simulink model "dx_hand_model_rai3"  (R2017b)
settings: Solver=ode3  StartTime=0.0  StopTime=inf  FixedStep=0.01  RelTol=1e-3  EnableMultiTasking=on
InitFcn:
  | cutFreq = 0.1; % T
  | sampleTime = 0.01;
  | filt = tf(1,[cutFreq 1]);
  | filt = c2d(filt,sampleTime);
  | 
  | cutFreq2 = 1;
  | filt2 = tf(1,[cutFreq2 1]);
  | filt2 = c2d(filt2,sampleTime);
  | 
  | update_param = 2;
  | 
  | ampliFactor = 1.60;
  | ampliFactorMiddle = 2.00;
  | ampliFactorDistal = 1;
  | 
  | % Set Hand Address
  | RightHandAddress = '10.24.4.91';
  | Verosim = '10.100.39.22'
  | LeftHandAddress = '10.24.4.90'
  | 
  | max_force = 12; % Newton
model workspace (MAT data in the model file):
  SL_ROS_VariableLengthArrays_MaxSizes.CommonInfo.ArrayTruncateAction = 'EmitWarning'
  SL_ROS_VariableLengthArrays_MaxSizes.MsgTypeMap = containers.Map
  SL_ROS_VariableLengthArrays_MaxSizes.MsgTypeMap.serialization.keys = {'std_msgs/Float32MultiArray'}
  SL_ROS_VariableLengthArrays_MaxSizes.MsgTypeMap.serialization.values{1}.PropertyName = 'Data'
  SL_ROS_VariableLengthArrays_MaxSizes.MsgTypeMap.serialization.values{1}.DataType = 'single'
  SL_ROS_VariableLengthArrays_MaxSizes.MsgTypeMap.serialization.values{1}.MaxLength = 2
  SL_ROS_VariableLengthArrays_MaxSizes.MsgTypeMap.serialization.uniformity = 0
  SL_ROS_VariableLengthArrays_MaxSizes.MsgTypeMap.serialization.keyType = 'char'
  SL_ROS_VariableLengthArrays_MaxSizes.MsgTypeMap.serialization.valueType = 'any'
libraries: robotlib x134, simulink_extras x28, simulink x16, dspnetwork x5, etargetslib x4
(part 1 of 19)
settings Model: Creator=Centauro  LastModifiedBy=exo-hand
settings DataIOCC: LimitDataPoints=on  SaveFormat=Array
settings OptimizationCC: PassReuseOutputArgsThreshold=0  MaxStackSize=64
settings DebuggingCC: ParameterTunabilityLossMsg=error  SFUnexpectedBacktrackingDiag=warning  SFNoUnconditionalDefaultTransitionDiag=warning  SFExecutionAtInitializationDiag=none
settings HardwareCC: ProdBitPerPointer=32  ProdBitPerSizeT=32  ProdBitPerPtrDiffT=32  ProdLargestAtomicFloat=None  ProdIntDivRoundTo=Undefined  ProdEndianess=Unspecified  ProdWordSize=32  ProdHWDeviceType=Generic->Unspecified (assume 32-bit Generic)  UseEmbeddedCoderFeatures=off
settings ModelReferenceCC: PropagateSignalLabelsOutOfModel=off
settings SFSimCC: MATLABDynamicMemAlloc=off
settings RTWCC: SystemTargetFile=ert.tlc  HardwareBoard=Robot Operating System (ROS)  TemplateMakefile=ert_default_tmf  GenerateReport=on  Toolchain=Catkin  LaunchReport=on  TargetLang=C++
settings CodeAppCC: ForceParamTrailComments=on  OperatorAnnotations=on
settings ERTTargetCC: ERTCustomFileBanners=off  SupportContinuousTime=on  SupportNonInlinedSFcns=on  RemoveResetFunc=off  ModelStepFunctionPrototypeControlCompliant=off
settings ConfigComp: CovMetricSettings=dw  CovHtmlReporting=on  CovSaveCumulativeToWorkspaceVar=on  CovSaveSingleToWorkspaceVar=on  CovExternalEMLEnable=off

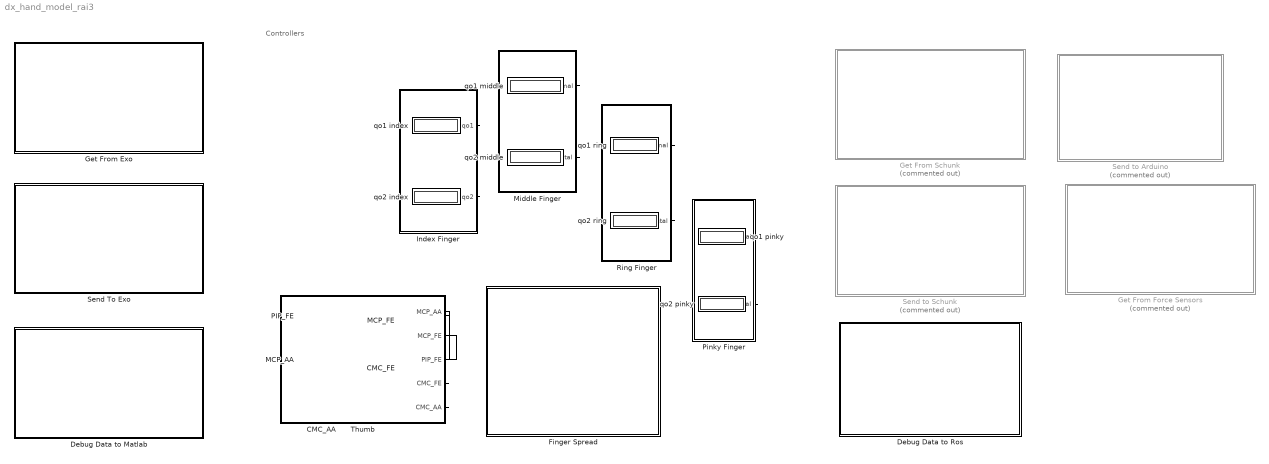
== system dx_hand_model_rai3 ==
  note: Controllers
  CMC_AA : Display
  CMC_FE : Display
  Debug Data to Matlab : Subsystem
  Debug Data to Ros : Subsystem
  Finger Spread : Subsystem
  Get From Exo : Subsystem
  Get From Force Sensors : Subsystem  Commented=on
  Get From Schunk : Subsystem  Commented=on
  Index Finger : Subsystem
  MCP_AA : Display
  MCP_FE : Display
  Middle Finger : Subsystem
  PIP_FE : Display
  Pinky Finger : Subsystem
  "Ring Finger " : Subsystem
  Send To Exo : Subsystem
  Send to Arduino : Subsystem  Commented=on
  Send to Schunk : Subsystem  Commented=on
  Thumb : Subsystem
  qo1 index : Display
  qo1 middle : Display
  qo1 pinky : Display
  qo1 ring : Display
  qo2 index : Display
  qo2 middle : Display
  qo2 pinky : Display
  qo2 ring : Display
  wires:
  Pinky Finger/1(proximal) -> qo1 pinky/1
  "Ring Finger "/1(proximal) -> qo1 ring/1
  Index Finger/2("qo2 ") -> qo2 index/1
  Index Finger/1("qo1 ") -> qo1 index/1
  Middle Finger/2(distal) -> qo2 middle/1
  Middle Finger/1(proximal) -> qo1 middle/1
  Thumb/1(MCP_AA) -> MCP_AA/1
  Thumb/2(MCP_FE) -> MCP_FE/1
  Thumb/4(CMC_FE) -> CMC_FE/1
  Thumb/3(PIP_FE) -> PIP_FE/1
  Thumb/5(CMC_AA) -> CMC_AA/1
  "Ring Finger "/2(distal) -> qo2 ring/1
  Pinky Finger/2(distal) -> qo2 pinky/1

== system dx_hand_model_rai3/Debug Data to Matlab ==
  Constant : Constant
  Constant1 : Constant  Value=0
  Manual Switch : ManualSwitch
  Mux : Mux  Inputs=20
  Thumb Exo Structure : Subsystem
  wires:
  Manual Switch/1 -> Thumb Exo Structure/Enable
  Constant/1 -> Manual Switch/2
  Constant1/1 -> Manual Switch/1
  [thumb_i] -> Mux/11
  [thumb_g2] -> Mux/9
  [thumb_c] -> Mux/3
  [thumb_d] -> Mux/4
  [thumb_f] -> Mux/7
  [thumb_f1] -> Mux/6
  [thumb_h] -> Mux/10
  [thumb_b] -> Mux/2
  Mux/1 -> Thumb Exo Structure/1(In1)
  [thumb_j] -> Mux/12
  [thumb_CMC] -> Mux/1
  [thumb_e] -> Mux/5
  [thumb_g1] -> Mux/8
  [thumb_MCP] -> Mux/13
  [thumb_K] -> Mux/14
  [thumb_PIP] -> Mux/15
  [thumb_K2] -> Mux/16
  [thumb_s1] -> Mux/17
  [thumb_l_meta] -> Mux/18
  [thumb_s2] -> Mux/19
  [thumb_l_dist] -> Mux/20

== system dx_hand_model_rai3/Debug Data to Ros ==
  Send : Subsystem
  Vector Concatenate : Concatenate  NumInputs=5
  Vector Concatenate1 : Concatenate  NumInputs=5
  wires:
  Vector Concatenate/1 -> Send/1(to_exo)
  Vector Concatenate1/1 -> Send/2(from_exo)
  [SetHandIndexForce] -> Vector Concatenate/2
  [SetHandRingForce] -> Vector Concatenate/4
  [SetHandThumbForce] -> Vector Concatenate/1
  [SetHandMiddleForce] -> Vector Concatenate/3
  [SetHandPinkyForce] -> Vector Concatenate/5
  [PinkyForce] -> Vector Concatenate1/5
  [RingForce] -> Vector Concatenate1/4
  [MiddleForce] -> Vector Concatenate1/3
  [IndexForce] -> Vector Concatenate1/2
  [ThumbForce] -> Vector Concatenate1/1

== system dx_hand_model_rai3/Finger Spread ==
  Constant : Constant  Value=0.0  OutDataTypeStr=single
  Constant1 : Constant  Value=0.15  OutDataTypeStr=single
  Display : Display
  MATLAB Function : MATLAB Function  TreatAsAtomicUnit=on
  Manual Switch : ManualSwitch  CurrentSetting=0
  Mux : Mux  Inputs=2
  Sum : Sum  Inputs=|++
  calibration1 : Subsystem
  tag scope: SchunkFingerSpread=global
  wires:
  [IndexSpreadRotPot] -> calibration1/1(In1), MATLAB Function/1(u)
  Constant/1 -> Manual Switch/2
  MATLAB Function/1(y) -> Manual Switch/1
  calibration1/1(Out1) -> Mux/2, MATLAB Function/2(calib)
  Mux/1 -> Display/1
  Manual Switch/1 -> Sum/1
  Sum/1 -> Mux/1, [SchunkFingerSpread]
  Constant1/1 -> Sum/2

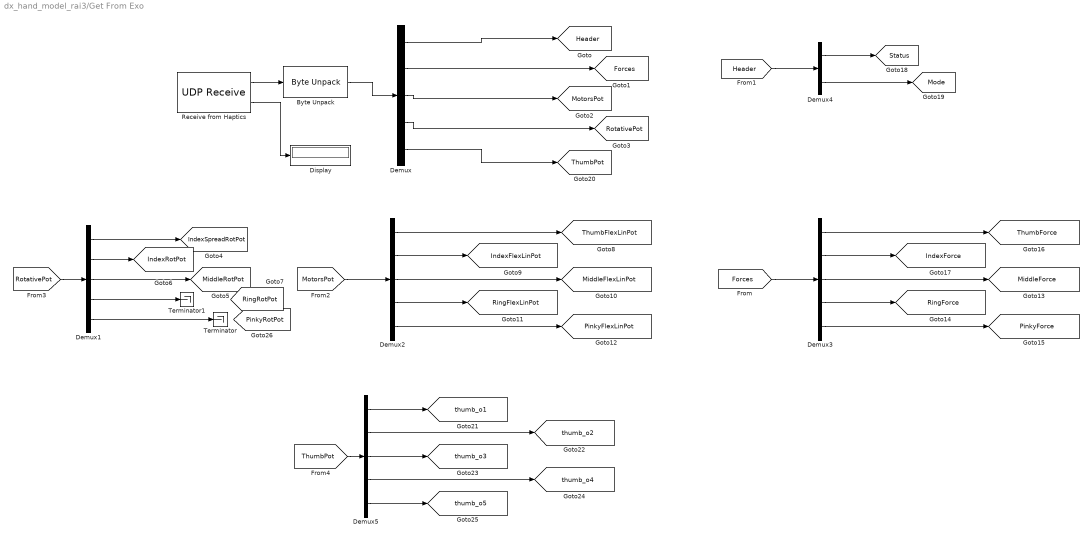
== system dx_hand_model_rai3/Get From Exo ==
  Byte Unpack : etargetslib/Byte Unpack  dimensions={[22]}  datatypes={'single'}  byteAlign=1
  Demux : Demux  Outputs=[2, 5, 5, 5,5]
  Demux{1..3,5} (4 alike) : Demux  Outputs=5
  Demux4 : Demux  Outputs=2
  Display : Display
  Receive from Haptics : dspnetwork/UDP Receive  localURL='0.0.0.0'  localPort=15001  remoteURL='0.0.0.0'  remotePort=-1  recvBufferSize=22*4  dims=22*4  signalDatatype=uint8  isVarSize=off  showBlockingTime=on  blockingTime=inf  sampletime=0.01  blockPlatform=HOST
      settings: SourceProductName=DSP System Toolbox  SourceProductBaseCode=DS
  Terminator : Terminator
  Terminator1 : Terminator
  tag scope: Forces=global, Header=global, IndexFlexLinPot=global, IndexForce=global, IndexRotPot=global, IndexSpreadRotPot=global, MiddleFlexLinPot=global, MiddleForce=global, MiddleRotPot=global, Mode=global, MotorsPot=global, PinkyFlexLinPot=global, PinkyForce=global, PinkyRotPot=global, RingFlexLinPot=global, RingForce=global, RingRotPot=global, RotativePot=global, Status=global, ThumbFlexLinPot=global, ThumbForce=global, ThumbPot=global, thumb_o1=global, thumb_o2=global, thumb_o3=global, thumb_o4=global, thumb_o5=global
  wires:
  Demux/3 -> [MotorsPot]
  Demux/1 -> [Header]
  Demux/4 -> [RotativePot]
  Demux/2 -> [Forces]
  Receive from Haptics/2 -> Display/1
  [RotativePot] -> Demux1/1
  Demux1/2 -> [IndexRotPot]
  Demux1/3 -> [MiddleRotPot]
  Demux1/4 -> Terminator1/1
  Demux1/5 -> Terminator/1
  Demux1/1 -> [IndexSpreadRotPot]
  Demux2/1 -> [ThumbFlexLinPot]
  Demux2/2 -> [IndexFlexLinPot]
  [MotorsPot] -> Demux2/1
  Demux2/3 -> [MiddleFlexLinPot]
  Demux2/4 -> [RingFlexLinPot]
  Demux2/5 -> [PinkyFlexLinPot]
  Demux3/1 -> [ThumbForce]
  Demux3/2 -> [IndexForce]
  [Forces] -> Demux3/1
  Demux3/3 -> [MiddleForce]
  Demux3/4 -> [RingForce]
  Demux3/5 -> [PinkyForce]
  [Header] -> Demux4/1
  Demux4/1 -> [Status]
  Demux4/2 -> [Mode]
  Byte Unpack/1 -> Demux/1
  Receive from Haptics/1 -> Byte Unpack/1
  Demux/5 -> [ThumbPot]
  [ThumbPot] -> Demux5/1
  Demux5/1 -> [thumb_o1]
  Demux5/2 -> [thumb_o2]
  Demux5/3 -> [thumb_o3]
  Demux5/4 -> [thumb_o4]
  Demux5/5 -> [thumb_o5]

== system dx_hand_model_rai3/Get From Force Sensors ==
  Currents : Subsystem

== system dx_hand_model_rai3/Get From Schunk ==
  Currents : Subsystem
  Get positions : Subsystem

== system dx_hand_model_rai3/Index Finger ==
  note: To Schunk
  note: To Exo
  Active : Subsystem
  Choose : Subsystem
  Display : Display
  Force : Subsystem
  Jacobian Calculation : Subsystem
  Pose Generator : Subsystem
  Position : Subsystem
  Pre-Proc : Subsystem
  Send Position : Subsystem
  setGain2 : Subsystem
  "qo1 " : Outport
  "qo2 " : Outport  Port=2
  tag scope: IndexForceReference=global
  wires:
  Pose Generator/1(Pose) -> Send Position/1(Pose), Jacobian Calculation/1(Pose)
  Pose Generator/2(Sensors) -> Jacobian Calculation/2(Sensor)
  Pose Generator/3("Measurements ") -> Jacobian Calculation/3(Measurements)
  Send Position/1(qo1) -> "qo1 "/1
  Send Position/2("qo2 ") -> "qo2 "/1
  Position/1(rate) -> Choose/1(pos)
  Force/1(Feedforward Force) -> Choose/2(force)
  Choose/1(out) -> setGain2/1(in)
  setGain2/1(out) -> Display/1, Active/1(in)
  Jacobian Calculation/1(Jac) -> Pre-Proc/1(in)
  Pre-Proc/1(out) -> Force/1(Jacobian), Position/1(Jacobian)
  Active/1(out) -> [IndexForceReference]

== system dx_hand_model_rai3/Middle Finger ==
  note: To Schunk
  note: To Exo
  Active : Subsystem
  Choose : Subsystem
  Demux : Demux  Outputs=8
  Display2 : Display
  Jacobian Calculation : Subsystem
  Pose Generator : Subsystem
  Position-Force Architecture : Subsystem
  Position-Position : Subsystem
  Pre-Proc : Subsystem
  Radians to Degrees : simulink_extras/Transformations/Radians to Degrees
  Radians to Degrees1 : simulink_extras/Transformations/Radians to Degrees
  setGain : Subsystem
  setGain1 : Subsystem
  setGain2 : Subsystem
  proximal : Outport
  distal : Outport  Port=2
  tag scope: MiddleForceReference=global, SchunkMiddleFingerDistal=global, SchunkMiddleFingerProximal=global
  wires:
  Demux/2 -> Radians to Degrees/1, setGain1/1(in)
  Pose Generator/1(Pose) -> Demux/1, Jacobian Calculation/1(Pose)
  Pose Generator/2(Sensors) -> Jacobian Calculation/2(Sensor)
  Pose Generator/3(Measurements) -> Jacobian Calculation/3(Measurements)
  Demux/1 -> Radians to Degrees1/1, setGain/1(in)
  Radians to Degrees1/1 -> proximal/1
  Radians to Degrees/1 -> distal/1
  Position-Force Architecture/1(Feedforward Force) -> Choose/2(force)
  Jacobian Calculation/1(Jacobian) -> Pre-Proc/1(in)
  Pre-Proc/1(out) -> Position-Position/1(Jacobian), Position-Force Architecture/1(Jacobian)
  setGain2/1(out) -> Display2/1, Active/1(in)
  Position-Position/1(rate) -> Choose/1(pos)
  setGain/1(out) -> [SchunkMiddleFingerProximal]
  setGain1/1(out) -> [SchunkMiddleFingerDistal]
  Choose/1(out) -> setGain2/1(in)
  Active/1(out) -> [MiddleForceReference]

== system dx_hand_model_rai3/Pinky Finger ==
  note: To Exo
  note: To Schunk
  Active : Subsystem
  Choose : Subsystem
  Choose_ : Subsystem
  Demux : Demux  Outputs=8
  Display2 : Display
  Gain Aggiustato : Gain  Gain=50/1024
  Gain1 : Gain  Gain=0.98/40
  Jacobian Calculation : Subsystem
  Pose Generator : Subsystem
  Position-Force Architecture : Subsystem
  Position-Position : Subsystem
  Pre-Proc : Subsystem
  Radians to Degrees : simulink_extras/Transformations/Radians to Degrees
  Radians to Degrees1 : simulink_extras/Transformations/Radians to Degrees
  setGain : Subsystem
  setGain1 : Subsystem
  setGain2 : Subsystem
  proximal : Outport
  distal : Outport  Port=2
  tag scope: PinkyForceReference=global, SchunkPinkyFinger=global, SchunkPinkyFingerDistal=global, SchunkPinkyFingerProximal=global
  wires:
  [PinkyFlexLinPot] -> Gain Aggiustato/1
  Gain1/1 -> Choose/2(empiric)
  Gain Aggiustato/1 -> Gain1/1
  Jacobian Calculation/1(Jacobian) -> Pre-Proc/1(in)
  Position-Force Architecture/1(Feedforward Force) -> Choose_/2(force)
  Pose Generator/2(Sensors) -> Jacobian Calculation/2(Sensor)
  Choose_/1(out) -> setGain2/1(in)
  Pose Generator/3(Measurements) -> Jacobian Calculation/3(Measurements)
  Demux/2 -> Radians to Degrees/1, setGain1/1(in)
  Position-Position/1(rate) -> Choose_/1(pos)
  Radians to Degrees/1 -> distal/1
  Radians to Degrees1/1 -> proximal/1
  setGain2/1(out) -> Display2/1, Active/1(in)
  setGain1/1(out) -> [SchunkPinkyFingerDistal]
  setGain/1(out) -> Choose/1(theoretical), [SchunkPinkyFingerProximal]
  Pre-Proc/1(out) -> Position-Position/1(Jacobian), Position-Force Architecture/1(Jacobian)
  Demux/1 -> Radians to Degrees1/1, setGain/1(in)
  Pose Generator/1(Pose) -> Demux/1, Jacobian Calculation/1(Pose)
  Active/1(out) -> [PinkyForceReference]
  Choose/1(out) -> [SchunkPinkyFinger]

== system dx_hand_model_rai3/Ring Finger  ==
  note: To Schunk
  note: To Exo
  Active : Subsystem
  Choose : Subsystem
  Choose_ : Subsystem
  Demux : Demux  Outputs=8
  Display2 : Display
  Gain Aggiustato : Gain  Gain=50/1024
  Gain1 : Gain  Gain=0.98/25
  Jacobian Calculation : Subsystem
  Pose Generator : Subsystem
  Position-Force Architecture : Subsystem
  Position-Position : Subsystem
  Pre-Proc : Subsystem
  Radians to Degrees : simulink_extras/Transformations/Radians to Degrees
  Radians to Degrees1 : simulink_extras/Transformations/Radians to Degrees
  setGain : Subsystem
  setGain1 : Subsystem
  setGain2 : Subsystem
  proximal : Outport
  distal : Outport  Port=2
  tag scope: RingForceReference=global, SchunkRingFinger=global, SchunkRingFingerDistal=global, SchunkRingFingerProximal=global
  wires:
  [RingFlexLinPot] -> Gain Aggiustato/1
  Gain Aggiustato/1 -> Gain1/1
  Gain1/1 -> Choose/2(empiric)
  Radians to Degrees1/1 -> proximal/1
  Position-Position/1(rate) -> Choose_/1(pos)
  Pose Generator/2(Sensors) -> Jacobian Calculation/2(Sensor)
  Choose_/1(out) -> setGain2/1(in)
  Radians to Degrees/1 -> distal/1
  setGain1/1(out) -> [SchunkRingFingerDistal]
  Pose Generator/1(Pose) -> Demux/1, Jacobian Calculation/1(Pose)
  setGain/1(out) -> Choose/1(theoretical), [SchunkRingFingerProximal]
  Position-Force Architecture/1(Feedforward Force) -> Choose_/2(force)
  Pose Generator/3(Measurements) -> Jacobian Calculation/3(Measurements)
  Pre-Proc/1(out) -> Position-Position/1(Jacobian), Position-Force Architecture/1(Jacobian)
  Demux/2 -> Radians to Degrees/1, setGain1/1(in)
  setGain2/1(out) -> Display2/1, Active/1(in)
  Jacobian Calculation/1(Jacobian) -> Pre-Proc/1(in)
  Demux/1 -> Radians to Degrees1/1, setGain/1(in)
  Active/1(out) -> [RingForceReference]
  Choose/1(out) -> [SchunkRingFinger]

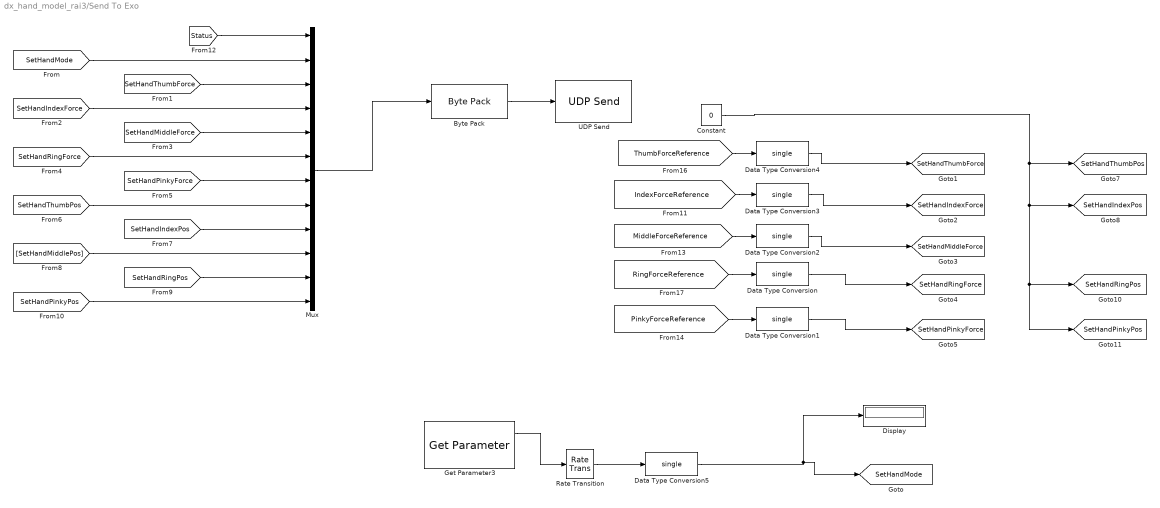
== system dx_hand_model_rai3/Send To Exo ==
  Byte Pack : etargetslib/Byte Pack  datatypes={'single'}  byteAlign=1
  Constant : Constant  Value=0  OutDataTypeStr=single
  Data Type Conversion{,1..5} (6 alike) : DataTypeConversion  OutDataTypeStr=single
  Display : Display
  Get Parameter3 : robotlib/Get Parameter  SourceLibraryInfo=This block requires Robotics System Toolbox  ParameterSource=Specify your own  ParameterName=/hand_exo/mode  ParameterType=double  ParameterMaxArrayLength=16  ParameterInitialValue=3.0  SampleTime=update_param  ShowErrorCodeOutput=on  ModelName=dx_hand_model_rai3  BlockId=ParamGet_dx_hand_model_rai3_2544
      settings: SourceProductName=Robotics System Toolbox  SourceProductBaseCode=RO
  Mux : Mux  Inputs=12
  Rate Transition : RateTransition
  UDP Send : dspnetwork/UDP Send  remoteURL=RightHandAddress  remotePort=12000  localURL='0.0.0.0'  localPortSource=Automatically determine  localPort=-1  sampletime=-1  blockPlatform=HOST  separateLengthPort=0
      settings: SourceProductName=DSP System Toolbox  SourceProductBaseCode=DS
  tag scope: SetHandIndexForce=global, SetHandIndexPos=global, SetHandMiddleForce=global, SetHandMode=global, SetHandPinkyForce=global, SetHandPinkyPos=global, SetHandRingForce=global, SetHandRingPos=global, SetHandThumbForce=global, SetHandThumbPos=global
  wires:
  Byte Pack/1 -> UDP Send/1
  [SetHandMode] -> Mux/2
  [SetHandThumbForce] -> Mux/3
  [SetHandIndexForce] -> Mux/4
  [SetHandRingForce] -> Mux/6
  [SetHandMiddleForce] -> Mux/5
  [SetHandPinkyForce] -> Mux/7
  [SetHandThumbPos] -> Mux/8
  [SetHandIndexPos] -> Mux/9
  [SetHandMiddlePos] -> Mux/10
  [SetHandRingPos] -> Mux/11
  [SetHandPinkyPos] -> Mux/12
  [Status] -> Mux/1
  [ThumbForceReference] -> Data Type Conversion4/1
  [RingForceReference] -> Data Type Conversion/1
  [PinkyForceReference] -> Data Type Conversion1/1
  [MiddleForceReference] -> Data Type Conversion2/1
  [IndexForceReference] -> Data Type Conversion3/1
  Constant/1 -> [SetHandThumbPos], [SetHandIndexPos], [SetHandRingPos], [SetHandPinkyPos]
  Mux/1 -> Byte Pack/1
  Data Type Conversion/1 -> [SetHandRingForce]
  Data Type Conversion1/1 -> [SetHandPinkyForce]
  Data Type Conversion2/1 -> [SetHandMiddleForce]
  Data Type Conversion3/1 -> [SetHandIndexForce]
  Data Type Conversion4/1 -> [SetHandThumbForce]
  Get Parameter3/1 -> Rate Transition/1
  Data Type Conversion5/1 -> [SetHandMode], Display/1
  Rate Transition/1 -> Data Type Conversion5/1

== system dx_hand_model_rai3/Send to Arduino ==
  Constant : Constant  Value=180
  Data Type Conversion2 : DataTypeConversion  OutDataTypeStr=uint8
  Display : Display
  Filt 4 : DiscreteTransferFcn  Numerator=filt.Numerator{1,1}  Denominator=filt.Denominator{1,1}  SampleTime=0.01
  Gain : Gain  Gain=180/60
  Radians to Degrees : simulink_extras/Transformations/Radians to Degrees
  Saturation : Saturate  UpperLimit=60  LowerLimit=0
  Sum : Sum  Inputs=|-+
  UDP Send : dspnetwork/UDP Send  remoteURL='10.24.4.20'  remotePort=9002  localURL='0.0.0.0'  localPortSource=Automatically determine  localPort=-1  sampletime=-1  blockPlatform=[]  separateLengthPort=0
      settings: SourceProductName=DSP System Toolbox  SourceProductBaseCode=DS
  wires:
  [SchunkIndexFingerProximal] -> Filt 4/1
  Filt 4/1 -> Radians to Degrees/1
  Radians to Degrees/1 -> Saturation/1
  Saturation/1 -> Gain/1
  Data Type Conversion2/1 -> Display/1, UDP Send/1
  Gain/1 -> Sum/1
  Sum/1 -> Data Type Conversion2/1
  Constant/1 -> Sum/2

== system dx_hand_model_rai3/Send to Schunk ==
  Enable : Subsystem  Commented=on
  Send data to Ros : Subsystem
  Signal Conditioning : Subsystem
  wires:
  Signal Conditioning/1(status) -> Send data to Ros/1(status)
  Signal Conditioning/3(data) -> Send data to Ros/2(data)

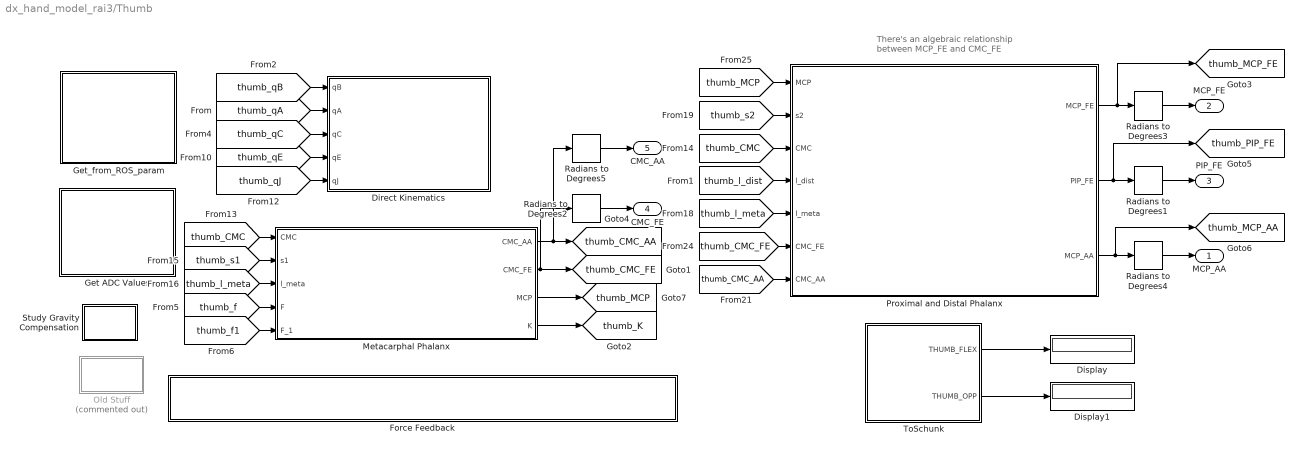
== system dx_hand_model_rai3/Thumb ==
  note: There's an algebraic relationship
      | between MCP_FE and CMC_FE
  Direct Kinematics : Subsystem
  Display : Display
  Display1 : Display
  Force Feedback : Subsystem
  Get ADC Values : Subsystem
  Get_from_ROS_param : Subsystem
  Metacarphal Phalanx : Subsystem
  Old Stuff : Subsystem  Commented=on
  Proximal and Distal Phalanx : Subsystem
  Radians to Degrees{1..5} (5 alike) : simulink_extras/Transformations/Radians to Degrees
  Study Gravity Compensation : Subsystem
  ToSchunk : Subsystem
  MCP_AA : Outport
  MCP_FE : Outport  Port=2
  PIP_FE : Outport  Port=3
  CMC_FE : Outport  Port=4
  CMC_AA : Outport  Port=5
  tag scope: thumb_CMC_AA=global, thumb_CMC_FE=global, thumb_K=global, thumb_MCP=global, thumb_MCP_AA=global, thumb_MCP_FE=global, thumb_PIP_FE=global
  wires:
  Metacarphal Phalanx/3(MCP) -> [thumb_MCP]
  Radians to Degrees3/1 -> MCP_FE/1
  Proximal and Distal Phalanx/1(MCP_FE) -> [thumb_MCP_FE], Radians to Degrees3/1
  Radians to Degrees4/1 -> MCP_AA/1
  [thumb_qA] -> Direct Kinematics/2(qA)
  [thumb_qB] -> Direct Kinematics/1(qB)
  [thumb_qC] -> Direct Kinematics/3(qC)
  [thumb_qE] -> Direct Kinematics/4(qE)
  [thumb_qJ] -> Direct Kinematics/5(qJ)
  [thumb_f] -> Metacarphal Phalanx/4(F)
  [thumb_f1] -> Metacarphal Phalanx/5(F_1)
  [thumb_CMC] -> Metacarphal Phalanx/1(CMC)
  [thumb_CMC] -> Proximal and Distal Phalanx/3(CMC)
  [thumb_s1] -> Metacarphal Phalanx/2(s1)
  [thumb_l_meta] -> Metacarphal Phalanx/3(l_meta)
  [thumb_l_dist] -> Proximal and Distal Phalanx/4(l_dist)
  [thumb_l_meta] -> Proximal and Distal Phalanx/5(l_meta)
  [thumb_s2] -> Proximal and Distal Phalanx/2(s2)
  [thumb_CMC_AA] -> Proximal and Distal Phalanx/7(CMC_AA)
  [thumb_CMC_FE] -> Proximal and Distal Phalanx/6(CMC_FE)
  [thumb_MCP] -> Proximal and Distal Phalanx/1("MCP ")
  Radians to Degrees1/1 -> PIP_FE/1
  Metacarphal Phalanx/4(K) -> [thumb_K]
  Metacarphal Phalanx/2(CMC_FE) -> [thumb_CMC_FE], Radians to Degrees2/1
  Metacarphal Phalanx/1("CMC_AA ") -> Radians to Degrees5/1, [thumb_CMC_AA]
  ToSchunk/1(THUMB_FLEX) -> Display/1
  ToSchunk/2(THUMB_OPP) -> Display1/1
  Proximal and Distal Phalanx/3(MCP_AA) -> [thumb_MCP_AA], Radians to Degrees4/1
  Radians to Degrees2/1 -> CMC_FE/1
  Radians to Degrees5/1 -> CMC_AA/1
  Proximal and Distal Phalanx/2(PIP_FE) -> [thumb_PIP_FE], Radians to Degrees1/1

== system dx_hand_model_rai3/Debug Data to Matlab/Thumb Exo Structure ==
  In1 : Inport
  Enable : EnablePort
  Data Type Conversion1 : DataTypeConversion  OutDataTypeStr=double
  To File : ToFile  Filename=exo_points.mat  MatrixName=points
  wires:
  In1/1 -> Data Type Conversion1/1
  Data Type Conversion1/1 -> To File/1

== system dx_hand_model_rai3/Debug Data to Ros/Send ==
  to_exo : Inport
  from_exo : Inport  Port=2
  Blank Message2 : robotlib/Blank Message  SourceLibraryInfo=This block requires Robotics System Toolbox  messageType=sensor_msgs/JointState  SampleTime=inf
      settings: SourceProductBaseCode=RO
  Data Type Conversion : DataTypeConversion  OutDataTypeStr=uint32
  MATLAB Function - Assign : MATLAB Function  TreatAsAtomicUnit=on
  Publish1 : robotlib/Publish  SourceLibraryInfo=This block requires Robotics System Toolbox  topicSource=Specify your own  topic=/hand_exo/debug  messageType=sensor_msgs/JointState  messageQueueLength=1
      settings: SourceProductBaseCode=RO
  wires:
  to_exo/1 -> MATLAB Function - Assign/2(to_exo)
  from_exo/1 -> MATLAB Function - Assign/3(from_exo)
  Blank Message2/1 -> MATLAB Function - Assign/1(blankMessage)
  Data Type Conversion/1 -> MATLAB Function - Assign/4(timeStamp)
  [Status] -> Data Type Conversion/1
  MATLAB Function - Assign/1(msg) -> Publish1/1

== system dx_hand_model_rai3/Finger Spread/calibration1 ==
  In1 : Inport
  Subsystem1 : Subsystem
  Out1 : Outport
  wires:
  [CalibrationSignal] -> Subsystem1/Enable
  In1/1 -> Subsystem1/1(In1)
  Subsystem1/1(Out1) -> Out1/1

== system dx_hand_model_rai3/Get From Force Sensors/Currents ==
  Bus Selector : BusSelector  OutputSignals=Position
  Current Finger Spread : Terminator
  Demux : Demux  Outputs=2
  Selector : Selector  IndexOptions=Index vector (dialog)  Indices=[1 2 3 4 5 6 7 8 9]  OutputSizes=1
  Subscribe : robotlib/Subscribe  SourceLibraryInfo=This block requires Robotics System Toolbox  topicSource=Select from ROS network  topic=/hand_exo/force_sensors  messageType=sensor_msgs/JointState  sampleTime=0.01  messageQueueLength=1
      settings: SourceProductBaseCode=RO
  Terminator : Terminator
  tag scope: CurrentIndexDistal=global, CurrentIndexProximal=global, CurrentMiddleDistal=global, CurrentMiddleProximal=global, CurrentPinky=global, CurrentRing=global
  wires:
  ? -> [CurrentMiddleProximal]
  ? -> Current Finger Spread/1
  Demux/2 -> [CurrentIndexDistal]
  Subscribe/2 -> Bus Selector/1
  ? -> [CurrentMiddleDistal]
  ? -> [CurrentPinky]
  Demux/1 -> [CurrentIndexProximal]
  Bus Selector/1 -> Selector/1  "<Position>"
  ? -> [CurrentRing]
  Selector/1 -> Demux/1
  Subscribe/1 -> Terminator/1

== system dx_hand_model_rai3/Get From Schunk/Currents ==
  Bus Selector : BusSelector  OutputSignals=Data
  Current Finger Spread : Terminator
  Demux : Demux  Outputs=9
  Selector : Selector  IndexOptions=Index vector (dialog)  Indices=[1 2 3 4 5 6 7 8 9]  OutputSizes=1
  Subscribe : robotlib/Subscribe  SourceLibraryInfo=This block requires Robotics System Toolbox  topicSource=Select from ROS network  topic=/svh_controller/channel_currents  messageType=std_msgs/Float64MultiArray  sampleTime=0.01  messageQueueLength=1
      settings: SourceProductBaseCode=RO
  Terminator : Terminator
  tag scope: CurrentIndexDistal=global, CurrentIndexProximal=global, CurrentMiddleDistal=global, CurrentMiddleProximal=global, CurrentPinky=global, CurrentRing=global, CurrentThumbFlex=global, CurrentThumbOpp=global
  wires:
  Demux/1 -> [CurrentThumbFlex]
  Demux/6 -> [CurrentMiddleProximal]
  Demux/9 -> Current Finger Spread/1
  Demux/3 -> [CurrentIndexDistal]
  Subscribe/2 -> Bus Selector/1
  Demux/5 -> [CurrentMiddleDistal]
  Demux/8 -> [CurrentPinky]
  Demux/4 -> [CurrentIndexProximal]
  Demux/2 -> [CurrentThumbOpp]
  Bus Selector/1 -> Selector/1  "<Data>"
  Demux/7 -> [CurrentRing]
  Selector/1 -> Demux/1
  Subscribe/1 -> Terminator/1

== system dx_hand_model_rai3/Get From Schunk/Get positions ==
  Bus Selector : BusSelector  OutputSignals=Position
  Bus Selector1 : BusSelector  OutputSignals=Effort
  Get Efforts : Subsystem
  Get Positions : Subsystem
  Subscribe1 : robotlib/Subscribe  SourceLibraryInfo=This block requires Robotics System Toolbox  topicSource=Select from ROS network  topic=/svh_controller/channel_feedback  messageType=sensor_msgs/JointState  sampleTime=0.01  messageQueueLength=1
      settings: SourceProductBaseCode=RO
  wires:
  Subscribe1/2 -> Bus Selector/1, Bus Selector1/1
  Bus Selector1/1 -> Get Efforts/1(<Effort>)  "<Effort>"
  Bus Selector/1 -> Get Positions/1(<Position>)  "<Position>"

== system dx_hand_model_rai3/Index Finger/Active ==
  in : Inport
  Constant : Constant  Value=0  OutDataTypeStr=single
  Data Type Conversion1 : DataTypeConversion  OutDataTypeStr=single
  Get Parameter3 : robotlib/Get Parameter  SourceLibraryInfo=This block requires Robotics System Toolbox  ParameterSource=Specify your own  ParameterName=/hand_exo/index/modes/ff_active  ParameterType=double  ParameterMaxArrayLength=16  ParameterInitialValue=1.0  SampleTime=update_param  ShowErrorCodeOutput=off  ModelName=dx_hand_model_rai3  BlockId=ParamGet_dx_hand_model_rai3_4854
      settings: SourceProductName=Robotics System Toolbox  SourceProductBaseCode=RO
  Rate Transition : RateTransition
  Switch : Switch  Criteria=u2 > Threshold
  out : Outport
  wires:
  Switch/1 -> out/1
  Data Type Conversion1/1 -> Switch/2
  Rate Transition/1 -> Data Type Conversion1/1
  Get Parameter3/1 -> Rate Transition/1
  in/1 -> Switch/1
  Constant/1 -> Switch/3

== system dx_hand_model_rai3/Index Finger/Choose ==
  pos : Inport
  force : Inport  Port=2
  Data Type Conversion1 : DataTypeConversion  OutDataTypeStr=single
  Get Parameter3 : robotlib/Get Parameter  SourceLibraryInfo=This block requires Robotics System Toolbox  ParameterSource=Specify your own  ParameterName=/hand_exo/index/modes/type  ParameterType=double  ParameterMaxArrayLength=16  ParameterInitialValue=1.0  SampleTime=update_param  ShowErrorCodeOutput=off  ModelName=dx_hand_model_rai3  BlockId=ParamGet_dx_hand_model_rai3_3562
      settings: SourceProductName=Robotics System Toolbox  SourceProductBaseCode=RO
  Rate Transition : RateTransition
  Switch : Switch  Criteria=u2 > Threshold
  out : Outport
  wires:
  Switch/1 -> out/1
  Data Type Conversion1/1 -> Switch/2
  Rate Transition/1 -> Data Type Conversion1/1
  Get Parameter3/1 -> Rate Transition/1
  force/1 -> Switch/3
  pos/1 -> Switch/1

== system dx_hand_model_rai3/Index Finger/Force ==
  Jacobian : Inport
  Classic_Static_Problem : MATLAB Function  TreatAsAtomicUnit=on
  Display6 : Display
  Optimized_Static_Problem : MATLAB Function  TreatAsAtomicUnit=on
  Position Force Basic Architecture : Subsystem
  Subsystem : Subsystem
  Feedforward Force : Outport
  wires:
  Position Force Basic Architecture/1(force_vec) -> Classic_Static_Problem/2(force_vector), Optimized_Static_Problem/2(force_vector)
  Jacobian/1 -> Classic_Static_Problem/1(Jcomponents), Optimized_Static_Problem/1(Jcomponents)
  Subsystem/1(J_out) -> Feedforward Force/1, Display6/1
  Optimized_Static_Problem/1(y) -> Subsystem/1(optim)
  Classic_Static_Problem/1(y) -> Subsystem/2(classic)

== system dx_hand_model_rai3/Index Finger/Jacobian Calculation ==
  Pose : Inport
  Sensor : Inport  Port=2
  Measurements : Inport  Port=3
  Data Type Conversion1 : DataTypeConversion  OutDataTypeStr=single
  Data Type Conversion2 : DataTypeConversion  OutDataTypeStr=single
  Display7 : Display
  Jacobian : MATLAB Function  TreatAsAtomicUnit=on  SystemSampleTime=0.01
  "Jacobian Optim " : MATLAB Function  TreatAsAtomicUnit=on  SystemSampleTime=0.01
  Manual Switch : ManualSwitch
  Unit Delay1 : UnitDelay  InitialCondition=-1  SampleTime=0.01
  Unit Delay3 : UnitDelay  InitialCondition=[0;2.3]  SampleTime=0.01
  Jac : Outport
  wires:
  Measurements/1 -> "Jacobian Optim "/3(measurements), Jacobian/3(measurements)
  Pose/1 -> "Jacobian Optim "/1(pose), Jacobian/1(pose)
  Sensor/1 -> "Jacobian Optim "/2(sensor), Jacobian/2(sensor)
  Jacobian/3(J22_ol) -> Unit Delay1/1
  Unit Delay3/1 -> Data Type Conversion2/1
  Data Type Conversion1/1 -> Jacobian/5(J22_old)
  Jacobian/2(q_next) -> Unit Delay3/1
  Unit Delay1/1 -> Data Type Conversion1/1
  Data Type Conversion2/1 -> Jacobian/4(q_pr)
  Jacobian/1(J) -> Manual Switch/2
  "Jacobian Optim "/1(J) -> Manual Switch/1
  Manual Switch/1 -> Jac/1, Display7/1

== system dx_hand_model_rai3/Index Finger/Pose Generator ==
  Angular Potentiometer : Subsystem
  Constant : Constant
  Constant3 : Constant  Value=0
  Display : Display
  Display1 : Display
  Display3 : Display
  Index Direct Kinematics : MATLAB Function  TreatAsAtomicUnit=on
  Manual Switch : ManualSwitch  CurrentSetting=0
  Mux1 : Mux  Inputs=2
  Parameters : Subsystem
  Parametri Dito : Subsystem
  Rate Transition : RateTransition
  Record : Subsystem
  Saturation2 : Saturate  UpperLimit=1000  LowerLimit=0
  Saturation3 : Saturate  UpperLimit=1000  LowerLimit=0
  Subsystem : Subsystem
  Pose : Outport
  Sensors : Outport  Port=2
  "Measurements " : Outport  Port=3
  wires:
  Index Direct Kinematics/1(y) -> Pose/1, Record/3(output)
  [IndexRotPot] -> Angular Potentiometer/1(ADC)
  Saturation2/1 -> Mux1/2
  Saturation3/1 -> Mux1/1
  Constant/1 -> Manual Switch/1
  Mux1/1 -> Sensors/1, Index Direct Kinematics/1(u), Record/1(input)
  Angular Potentiometer/1(Deg) -> Display3/1
  Manual Switch/1 -> Record/Enable
  Constant3/1 -> Manual Switch/2
  Parameters/1("to_dir_kin ") -> Index Direct Kinematics/2(measurements), "Measurements "/1, Record/2(param)
  [IndexFlexLinPot] -> Subsystem/1(ADC)
  Angular Potentiometer/2(Rad) -> Saturation2/1, Display1/1
  Subsystem/1("lx ") -> Display/1, Saturation3/1
  Parametri Dito/1(Par) -> Rate Transition/1
  Rate Transition/1 -> Parameters/1(In1)

== system dx_hand_model_rai3/Index Finger/Position ==
  Jacobian : Inport
  Classic_Static_Problem : MATLAB Function  TreatAsAtomicUnit=on
  Discrete Derivative{,1..3} (4 alike) : simulink/Discrete/Discrete Derivative  gainval=1.0  ICPrevScaledInput=0.0  OutMin=[]  OutMax=[]  OutDataType=fixdt(1, 16)  OutScaling=2^-10  DoSatur=off
  Mux : Mux  Inputs=2
  Mux1 : Mux  Inputs=2
  Optimized_Static_Problem : MATLAB Function  TreatAsAtomicUnit=on
  Pre-Proc : Subsystem
  Saturation3 : Saturate  UpperLimit=0.80  LowerLimit=0
  Saturation4 : Saturate  UpperLimit=1.33  LowerLimit=0
  Sum{,1,3..4} (4 alike) : Sum  Inputs=|+-
  Sum2 : Sum  Inputs=|++
  active : Subsystem
  active1 : Subsystem
  setGain : Subsystem
  "setGain " : Subsystem
  setGain 1 : Subsystem
  setGain 2 : Subsystem
  rate : Outport
  wires:
  [act_IndexProxi] -> Discrete Derivative2/1, Sum/1
  Sum/1 -> setGain/1(in)
  "setGain "/1(out) -> Mux/2
  setGain/1(out) -> Mux/1
  [SchunkIndexFingerDistal] -> Saturation4/1
  Mux/1 -> Sum2/1
  Mux1/1 -> Sum2/2
  Sum2/1 -> Optimized_Static_Problem/2(force_vector), Classic_Static_Problem/2(operational_space)
  [SchunkIndexFingerProximal] -> Saturation3/1
  Saturation3/1 -> Discrete Derivative/1, Sum/2
  Saturation4/1 -> Sum1/2, Discrete Derivative1/1
  [act_IndexDistal] -> Discrete Derivative3/1, Sum1/1
  Jacobian/1 -> Optimized_Static_Problem/1(Jcomponents), Classic_Static_Problem/1(Jcomponents)
  Sum1/1 -> "setGain "/1(in)
  Discrete Derivative2/1 -> active/1(in)
  Discrete Derivative3/1 -> active1/1(in)
  Sum3/1 -> setGain 1/1(in)
  Sum4/1 -> setGain 2/1(in)
  setGain 1/1(out) -> Mux1/1
  setGain 2/1(out) -> Mux1/2
  Optimized_Static_Problem/1(y) -> Pre-Proc/1(yes)
  Classic_Static_Problem/1(rate) -> Pre-Proc/2(no)
  Pre-Proc/1(out) -> rate/1
  Discrete Derivative/1 -> Sum3/2
  Discrete Derivative1/1 -> Sum4/2
  active/1(out) -> Sum3/1
  active1/1(out) -> Sum4/1

== system dx_hand_model_rai3/Index Finger/Pre-Proc ==
  in : Inport
  Data Type Conversion1 : DataTypeConversion  OutDataTypeStr=single
  Data Type Conversion2 : DataTypeConversion  OutDataTypeStr=single
  Filt 4 : DiscreteTransferFcn  Numerator=filt2.Numerator{1,1}  Denominator=filt2.Denominator{1,1}  SampleTime=0.01
  Get Parameter3 : robotlib/Get Parameter  SourceLibraryInfo=This block requires Robotics System Toolbox  ParameterSource=Specify your own  ParameterName=/hand_exo/index/j_f  ParameterType=double  ParameterMaxArrayLength=16  ParameterInitialValue=1.0  SampleTime=update_param  ShowErrorCodeOutput=on  ModelName=dx_hand_model_rai3  BlockId=ParamGet_dx_hand_model_rai3_3238
      settings: SourceProductName=Robotics System Toolbox  SourceProductBaseCode=RO
  "IsNan " : MATLAB Function  TreatAsAtomicUnit=on
  Memory : Memory  InitialCondition=[0,0,0,0]
  Rate Transition : RateTransition
  Switch : Switch  Criteria=u2 > Threshold
  out : Outport
  wires:
  Get Parameter3/1 -> Rate Transition/1
  Rate Transition/1 -> Data Type Conversion1/1
  Data Type Conversion1/1 -> Switch/2
  Filt 4/1 -> Switch/1
  Switch/1 -> out/1
  "IsNan "/1(J) -> Switch/3, Filt 4/1, Memory/1
  Memory/1 -> Data Type Conversion2/1
  Data Type Conversion2/1 -> "IsNan "/2(J_k1)
  in/1 -> "IsNan "/1(Jin)

== system dx_hand_model_rai3/Index Finger/Send Position ==
  Pose : Inport
  Demux3 : Demux  Outputs=8
  Radians to Degrees : simulink_extras/Transformations/Radians to Degrees
  Radians to Degrees1 : simulink_extras/Transformations/Radians to Degrees
  setGain : Subsystem
  setGain1 : Subsystem
  qo1 : Outport
  "qo2 " : Outport  Port=2
  tag scope: SchunkIndexFingerDistal=global, SchunkIndexFingerProximal=global
  wires:
  Radians to Degrees1/1 -> "qo2 "/1
  Demux3/2 -> setGain1/1(in), Radians to Degrees1/1
  Demux3/1 -> setGain/1(in), Radians to Degrees/1
  Radians to Degrees/1 -> qo1/1
  Pose/1 -> Demux3/1
  setGain/1(out) -> [SchunkIndexFingerProximal]
  setGain1/1(out) -> [SchunkIndexFingerDistal]

== system dx_hand_model_rai3/Index Finger/setGain2 ==
  in : Inport
  Data Type Conversion1 : DataTypeConversion  OutDataTypeStr=single
  Get Parameter3 : robotlib/Get Parameter  SourceLibraryInfo=This block requires Robotics System Toolbox  ParameterSource=Specify your own  ParameterName=/hand_exo/index/modes/saturator  ParameterType=double  ParameterMaxArrayLength=16  ParameterInitialValue=-1.0  SampleTime=update_param  ShowErrorCodeOutput=off  ModelName=dx_hand_model_rai3  BlockId=ParamGet_dx_hand_model_rai3_3507
      settings: SourceProductName=Robotics System Toolbox  SourceProductBaseCode=RO
  Rate Transition : RateTransition
  Saturation1 : Saturate  UpperLimit=max_force  LowerLimit=-max_force
  Saturation2 : Saturate  UpperLimit=0  LowerLimit=-max_force
  Switch : Switch  Criteria=u2 > Threshold
  out : Outport
  wires:
  Switch/1 -> out/1
  Data Type Conversion1/1 -> Switch/2
  Rate Transition/1 -> Data Type Conversion1/1
  Get Parameter3/1 -> Rate Transition/1
  in/1 -> Saturation1/1, Saturation2/1
  Saturation1/1 -> Switch/1
  Saturation2/1 -> Switch/3

== system dx_hand_model_rai3/Middle Finger/Active ==
  in : Inport
  Constant : Constant  Value=0  OutDataTypeStr=single
  Data Type Conversion1 : DataTypeConversion  OutDataTypeStr=single
  Get Parameter3 : robotlib/Get Parameter  SourceLibraryInfo=This block requires Robotics System Toolbox  ParameterSource=Specify your own  ParameterName=/hand_exo/middle/modes/ff_active  ParameterType=double  ParameterMaxArrayLength=16  ParameterInitialValue=1.0  SampleTime=update_param  ShowErrorCodeOutput=off  ModelName=dx_hand_model_rai3  BlockId=ParamGet_dx_hand_model_rai3_4871
      settings: SourceProductName=Robotics System Toolbox  SourceProductBaseCode=RO
  Rate Transition : RateTransition
  Switch : Switch  Criteria=u2 > Threshold
  out : Outport
  wires:
  Switch/1 -> out/1
  Data Type Conversion1/1 -> Switch/2
  Rate Transition/1 -> Data Type Conversion1/1
  Get Parameter3/1 -> Rate Transition/1
  in/1 -> Switch/1
  Constant/1 -> Switch/3

== system dx_hand_model_rai3/Middle Finger/Choose ==
  pos : Inport
  force : Inport  Port=2
  Data Type Conversion1 : DataTypeConversion  OutDataTypeStr=single
  Get Parameter3 : robotlib/Get Parameter  SourceLibraryInfo=This block requires Robotics System Toolbox  ParameterSource=Specify your own  ParameterName=/hand_exo/middle/modes/type  ParameterType=double  ParameterMaxArrayLength=16  ParameterInitialValue=1.0  SampleTime=update_param  ShowErrorCodeOutput=off  ModelName=dx_hand_model_rai3  BlockId=ParamGet_dx_hand_model_rai3_3550
      settings: SourceProductName=Robotics System Toolbox  SourceProductBaseCode=RO
  Rate Transition : RateTransition
  Switch : Switch  Criteria=u2 > Threshold
  out : Outport
  wires:
  Switch/1 -> out/1
  Data Type Conversion1/1 -> Switch/2
  Rate Transition/1 -> Data Type Conversion1/1
  Get Parameter3/1 -> Rate Transition/1
  force/1 -> Switch/3
  pos/1 -> Switch/1

== system dx_hand_model_rai3/Middle Finger/Jacobian Calculation ==
  note: this jacobian has all lenght expressed in meters
  note: this jacobian has all lenght expressed in mm
  Pose : Inport
  Sensor : Inport  Port=2
  Measurements : Inport  Port=3
  Data Type Conversion1 : DataTypeConversion  OutDataTypeStr=single
  Data Type Conversion2 : DataTypeConversion  OutDataTypeStr=single
  Display1 : Display
  Display7 : Display
  Manual Switch : ManualSwitch
  Middle Jacobian : MATLAB Function  TreatAsAtomicUnit=on  SystemSampleTime=0.01
  "Middle Jacobian " : MATLAB Function  TreatAsAtomicUnit=on  SystemSampleTime=0.01
  Unit Delay1 : UnitDelay  InitialCondition=-1  SampleTime=0.01
  Unit Delay3 : UnitDelay  InitialCondition=[0;2.3]  SampleTime=0.01
  Jacobian : Outport
  wires:
  Middle Jacobian/1(JTcomp) -> Manual Switch/2, Display7/1
  Data Type Conversion1/1 -> Middle Jacobian/5(J22_old)
  Middle Jacobian/2(q_next) -> Unit Delay3/1
  Data Type Conversion2/1 -> Middle Jacobian/4(q_pr)
  Middle Jacobian/3(J22_ol) -> Unit Delay1/1
  Unit Delay3/1 -> Data Type Conversion2/1
  Unit Delay1/1 -> Data Type Conversion1/1
  Measurements/1 -> "Middle Jacobian "/3(measurements), Middle Jacobian/3(measurements)
  Sensor/1 -> "Middle Jacobian "/2(sensor), Middle Jacobian/2(sensor)
  "Middle Jacobian "/1(JTcomp) -> Display1/1, Manual Switch/1
  Pose/1 -> "Middle Jacobian "/1(pose), Middle Jacobian/1(pose)
  Manual Switch/1 -> Jacobian/1

== system dx_hand_model_rai3/Middle Finger/Pose Generator ==
  Angular Potentiometer : Subsystem
  Constant : Constant
  Constant3 : Constant  Value=0
  Display : Display
  Display1 : Display
  Display3 : Display
  Filtro : Subsystem  Commented=on
  Linear Potentiometer : Subsystem
  Manual Switch : ManualSwitch  CurrentSetting=0
  Middle Direct Kinematics : MATLAB Function  TreatAsAtomicUnit=on
  Mux1 : Mux  Inputs=2
  Parameters : Subsystem
  Parametri Dito : Subsystem
  Rate Transition : RateTransition
  Record : Subsystem
  Saturation2 : Saturate  UpperLimit=1000  LowerLimit=0
  Saturation3 : Saturate  UpperLimit=1000  LowerLimit=0
  Pose : Outport
  Sensors : Outport  Port=2
  Measurements : Outport  Port=3
  wires:
  Middle Direct Kinematics/1(y) -> Pose/1, Record/3(output)
  Manual Switch/1 -> Record/Enable
  Angular Potentiometer/1(Deg) -> Display3/1
  [MiddleRotPot] -> Angular Potentiometer/1(ADC)
  [MiddleFlexLinPot] -> Linear Potentiometer/1(ADC)
  Saturation2/1 -> Mux1/1
  Constant/1 -> Manual Switch/1
  Constant3/1 -> Manual Switch/2
  Angular Potentiometer/2(Rad) -> Display1/1, Saturation3/1
  Linear Potentiometer/1(mm) -> Display/1, Saturation2/1
  Mux1/1 -> Sensors/1, Record/1(input), Middle Direct Kinematics/1(u)
  Saturation3/1 -> Mux1/2
  Parameters/1(to Direct Kin) -> Middle Direct Kinematics/2(measurements), Measurements/1, Record/2(param)
  Parametri Dito/1(Par_5) -> Rate Transition/1
  Rate Transition/1 -> Parameters/1(Par5)

== system dx_hand_model_rai3/Middle Finger/Position-Force Architecture ==
  Jacobian : Inport
  Classic_Static_Problem : MATLAB Function  TreatAsAtomicUnit=on
  Display6 : Display
  Optimized_Static_Problem : MATLAB Function  TreatAsAtomicUnit=on
  Position Force Basic Architecture : Subsystem
  Subsystem : Subsystem
  Feedforward Force : Outport
  wires:
  Position Force Basic Architecture/1(force_vec) -> Classic_Static_Problem/2(force_vector), Optimized_Static_Problem/2(force_vector)
  Jacobian/1 -> Classic_Static_Problem/1(Jcomponents), Optimized_Static_Problem/1(Jcomponents)
  Subsystem/1(J_out) -> Feedforward Force/1, Display6/1
  Optimized_Static_Problem/1(y) -> Subsystem/1(optim)
  Classic_Static_Problem/1(y) -> Subsystem/2(classic)

== system dx_hand_model_rai3/Middle Finger/Position-Position ==
  Jacobian : Inport
  Classic_Static_Problem : MATLAB Function  TreatAsAtomicUnit=on
  Discrete Derivative{,1..3} (4 alike) : simulink/Discrete/Discrete Derivative  gainval=1.0  ICPrevScaledInput=0.0  OutMin=[]  OutMax=[]  OutDataType=fixdt(1, 16)  OutScaling=2^-10  DoSatur=off
  Mux : Mux  Inputs=2
  Mux1 : Mux  Inputs=2
  Optimized_Static_Problem : MATLAB Function  TreatAsAtomicUnit=on
  Pre-Proc : Subsystem
  Saturation3 : Saturate  UpperLimit=0.80  LowerLimit=0
  Saturation4 : Saturate  UpperLimit=1.33  LowerLimit=0
  Sum{,1,3..4} (4 alike) : Sum  Inputs=|+-
  Sum2 : Sum  Inputs=|++
  active : Subsystem
  active1 : Subsystem
  setGain : Subsystem
  "setGain " : Subsystem
  setGain 1 : Subsystem
  setGain 2 : Subsystem
  rate : Outport
  wires:
  [act_MiddleProxi] -> Discrete Derivative2/1, Sum/1
  Sum/1 -> setGain/1(in)
  "setGain "/1(out) -> Mux/2
  setGain/1(out) -> Mux/1
  [SchunkMiddleFingerDistal] -> Saturation4/1
  Mux/1 -> Sum2/1
  Mux1/1 -> Sum2/2
  Sum2/1 -> Optimized_Static_Problem/2(force_vector), Classic_Static_Problem/2(operational_space)
  [SchunkMiddleFingerProximal] -> Saturation3/1
  Saturation3/1 -> Sum/2, Discrete Derivative/1
  Saturation4/1 -> Sum1/2, Discrete Derivative1/1
  [act_MiddleDistal] -> Discrete Derivative3/1, Sum1/1
  Jacobian/1 -> Optimized_Static_Problem/1(Jcomponents), Classic_Static_Problem/1(Jcomponents)
  Sum1/1 -> "setGain "/1(in)
  Sum3/1 -> setGain 1/1(in)
  Sum4/1 -> setGain 2/1(in)
  setGain 1/1(out) -> Mux1/1
  setGain 2/1(out) -> Mux1/2
  Optimized_Static_Problem/1(y) -> Pre-Proc/1(yes)
  Classic_Static_Problem/1(rate) -> Pre-Proc/2(no)
  Pre-Proc/1(out) -> rate/1
  Discrete Derivative/1 -> Sum3/2
  Discrete Derivative1/1 -> Sum4/2
  Discrete Derivative2/1 -> active/1(in)
  active/1(out) -> Sum3/1
  Discrete Derivative3/1 -> active1/1(in)
  active1/1(out) -> Sum4/1

== system dx_hand_model_rai3/Middle Finger/Pre-Proc ==
  in : Inport
  Data Type Conversion1 : DataTypeConversion  OutDataTypeStr=single
  Data Type Conversion2 : DataTypeConversion  OutDataTypeStr=single
  Filt 4 : DiscreteTransferFcn  Numerator=filt2.Numerator{1,1}  Denominator=filt2.Denominator{1,1}  SampleTime=0.01
  Get Parameter3 : robotlib/Get Parameter  SourceLibraryInfo=This block requires Robotics System Toolbox  ParameterSource=Specify your own  ParameterName=/hand_exo/middle/j_f  ParameterType=double  ParameterMaxArrayLength=16  ParameterInitialValue=1.0  SampleTime=update_param  ShowErrorCodeOutput=on  ModelName=dx_hand_model_rai3  BlockId=ParamGet_dx_hand_model_rai3_3245
      settings: SourceProductName=Robotics System Toolbox  SourceProductBaseCode=RO
  "IsNan " : MATLAB Function  TreatAsAtomicUnit=on
  Memory : Memory  InitialCondition=[0,0,0,0]
  Rate Transition : RateTransition
  Switch : Switch  Criteria=u2 > Threshold
  out : Outport
  wires:
  Get Parameter3/1 -> Rate Transition/1
  Rate Transition/1 -> Data Type Conversion1/1
  Data Type Conversion1/1 -> Switch/2
  Filt 4/1 -> Switch/1
  Switch/1 -> out/1
  Memory/1 -> Data Type Conversion2/1
  in/1 -> "IsNan "/1(Jin)
  Data Type Conversion2/1 -> "IsNan "/2(J_k1)
  "IsNan "/1(J) -> Switch/3, Filt 4/1, Memory/1

== system dx_hand_model_rai3/Middle Finger/setGain ==
  in : Inport
  Data Type Conversion1 : DataTypeConversion  OutDataTypeStr=single
  Get Parameter3 : robotlib/Get Parameter  SourceLibraryInfo=This block requires Robotics System Toolbox  ParameterSource=Specify your own  ParameterName=/hand_exo/middle/schunk_gains/prox  ParameterType=double  ParameterMaxArrayLength=16  ParameterInitialValue=1.0  SampleTime=update_param  ShowErrorCodeOutput=off  ModelName=dx_hand_model_rai3  BlockId=ParamGet_dx_hand_model_rai3_3405
      settings: SourceProductName=Robotics System Toolbox  SourceProductBaseCode=RO
  Product : Product
  Rate Transition : RateTransition
  out : Outport
  wires:
  Product/1 -> out/1
  Data Type Conversion1/1 -> Product/1
  in/1 -> Product/2
  Rate Transition/1 -> Data Type Conversion1/1
  Get Parameter3/1 -> Rate Transition/1

== system dx_hand_model_rai3/Middle Finger/setGain1 ==
  in : Inport
  Data Type Conversion1 : DataTypeConversion  OutDataTypeStr=single
  Get Parameter3 : robotlib/Get Parameter  SourceLibraryInfo=This block requires Robotics System Toolbox  ParameterSource=Specify your own  ParameterName=/hand_exo/middle/schunk_gains/dist  ParameterType=double  ParameterMaxArrayLength=16  ParameterInitialValue=1.0  SampleTime=update_param  ShowErrorCodeOutput=off  ModelName=dx_hand_model_rai3  BlockId=ParamGet_dx_hand_model_rai3_3412
      settings: SourceProductName=Robotics System Toolbox  SourceProductBaseCode=RO
  Product : Product
  Rate Transition : RateTransition
  out : Outport
  wires:
  Product/1 -> out/1
  Data Type Conversion1/1 -> Product/1
  in/1 -> Product/2
  Rate Transition/1 -> Data Type Conversion1/1
  Get Parameter3/1 -> Rate Transition/1

== system dx_hand_model_rai3/Middle Finger/setGain2 ==
  in : Inport
  Data Type Conversion1 : DataTypeConversion  OutDataTypeStr=single
  Get Parameter3 : robotlib/Get Parameter  SourceLibraryInfo=This block requires Robotics System Toolbox  ParameterSource=Specify your own  ParameterName=/hand_exo/middle/modes/saturator  ParameterType=double  ParameterMaxArrayLength=16  ParameterInitialValue=-1.0  SampleTime=update_param  ShowErrorCodeOutput=off  ModelName=dx_hand_model_rai3  BlockId=ParamGet_dx_hand_model_rai3_3498
      settings: SourceProductName=Robotics System Toolbox  SourceProductBaseCode=RO
  Rate Transition : RateTransition
  Saturation1 : Saturate  UpperLimit=max_force  LowerLimit=-max_force
  Saturation2 : Saturate  UpperLimit=0  LowerLimit=-max_force
  Switch : Switch  Criteria=u2 > Threshold
  out : Outport
  wires:
  Switch/1 -> out/1
  Data Type Conversion1/1 -> Switch/2
  Rate Transition/1 -> Data Type Conversion1/1
  Get Parameter3/1 -> Rate Transition/1
  in/1 -> Saturation1/1, Saturation2/1
  Saturation1/1 -> Switch/1
  Saturation2/1 -> Switch/3

== system dx_hand_model_rai3/Pinky Finger/Active ==
  in : Inport
  Constant : Constant  Value=0  OutDataTypeStr=single
  Data Type Conversion1 : DataTypeConversion  OutDataTypeStr=single
  Get Parameter3 : robotlib/Get Parameter  SourceLibraryInfo=This block requires Robotics System Toolbox  ParameterSource=Specify your own  ParameterName=/hand_exo/pinky/modes/ff_active  ParameterType=double  ParameterMaxArrayLength=16  ParameterInitialValue=1.0  SampleTime=update_param  ShowErrorCodeOutput=off  ModelName=dx_hand_model_rai3  BlockId=ParamGet_dx_hand_model_rai3_4887
      settings: SourceProductName=Robotics System Toolbox  SourceProductBaseCode=RO
  Rate Transition : RateTransition
  Switch : Switch  Criteria=u2 > Threshold
  out : Outport
  wires:
  Switch/1 -> out/1
  Data Type Conversion1/1 -> Switch/2
  Rate Transition/1 -> Data Type Conversion1/1
  Get Parameter3/1 -> Rate Transition/1
  in/1 -> Switch/1
  Constant/1 -> Switch/3

== system dx_hand_model_rai3/Pinky Finger/Choose ==
  theoretical : Inport
  empiric : Inport  Port=2
  Data Type Conversion1 : DataTypeConversion  OutDataTypeStr=single
  Get Parameter3 : robotlib/Get Parameter  SourceLibraryInfo=This block requires Robotics System Toolbox  ParameterSource=Specify your own  ParameterName=/hand_exo/pinky/modes/theor  ParameterType=double  ParameterMaxArrayLength=16  ParameterInitialValue=-1.0  SampleTime=update_param  ShowErrorCodeOutput=off  ModelName=dx_hand_model_rai3  BlockId=ParamGet_dx_hand_model_rai3_4895
      settings: SourceProductName=Robotics System Toolbox  SourceProductBaseCode=RO
  Rate Transition : RateTransition
  Switch : Switch  Criteria=u2 > Threshold
  out : Outport
  wires:
  Switch/1 -> out/1
  Data Type Conversion1/1 -> Switch/2
  Rate Transition/1 -> Data Type Conversion1/1
  Get Parameter3/1 -> Rate Transition/1
  empiric/1 -> Switch/3
  theoretical/1 -> Switch/1

== system dx_hand_model_rai3/Pinky Finger/Choose_ ==
  pos : Inport
  force : Inport  Port=2
  Data Type Conversion1 : DataTypeConversion  OutDataTypeStr=single
  Get Parameter3 : robotlib/Get Parameter  SourceLibraryInfo=This block requires Robotics System Toolbox  ParameterSource=Specify your own  ParameterName=/hand_exo/pinky/modes/type  ParameterType=double  ParameterMaxArrayLength=16  ParameterInitialValue=1.0  SampleTime=update_param  ShowErrorCodeOutput=off  ModelName=dx_hand_model_rai3  BlockId=ParamGet_dx_hand_model_rai3_4579
      settings: SourceProductName=Robotics System Toolbox  SourceProductBaseCode=RO
  Rate Transition : RateTransition
  Switch : Switch  Criteria=u2 > Threshold
  out : Outport
  wires:
  Switch/1 -> out/1
  Data Type Conversion1/1 -> Switch/2
  Rate Transition/1 -> Data Type Conversion1/1
  Get Parameter3/1 -> Rate Transition/1
  force/1 -> Switch/3
  pos/1 -> Switch/1
